simulink model "Controller"  (R2015b)
settings: Solver=FixedStepAuto  StartTime=0.0  StopTime=inf  FixedStep=0.1  RelTol=1e-3
InitFcn:
  | robotics.ros.createSimulinkBus(gcs);
model workspace (MAT data in the model file):
  SL_ROS_VariableLengthArrays_MaxSizes : struct (value not decoded)
undefined symbols (not defined in the file or in its folder): DiscIntNeverNeededParam
libraries: robotlib x66, simulink x7, dspsrcs4 x6
(part 2 of 2)

== system Controller/toPWM/Enable thrusters  ==
  Get Parameter : robotlib/Get Parameter  SourceLibraryInfo=This block requires Robotics System Toolbox  ParameterSource=Specify your own  ParameterName=/matlab_controller/enable_thruster1  ParameterType=boolean  ParameterInitialValue=1  SampleTime=-1  ShowErrorCodeOutput=off  ModelName=Controller_without_ref  BlockId=ParamGet_Controller_without_ref_858
  Get Parameter1 : robotlib/Get Parameter  SourceLibraryInfo=This block requires Robotics System Toolbox  ParameterSource=Specify your own  ParameterName=/matlab_controller/enable_thruster2  ParameterType=boolean  ParameterInitialValue=1  SampleTime=-1  ShowErrorCodeOutput=off  ModelName=Controller_without_ref  BlockId=ParamGet_Controller_without_ref_861
  Get Parameter2 : robotlib/Get Parameter  SourceLibraryInfo=This block requires Robotics System Toolbox  ParameterSource=Specify your own  ParameterName=/matlab_controller/enable_thruster3  ParameterType=boolean  ParameterInitialValue=1  SampleTime=-1  ShowErrorCodeOutput=off  ModelName=Controller_without_ref  BlockId=ParamGet_Controller_without_ref_862
  Get Parameter3 : robotlib/Get Parameter  SourceLibraryInfo=This block requires Robotics System Toolbox  ParameterSource=Specify your own  ParameterName=/matlab_controller/enable_thruster4  ParameterType=boolean  ParameterInitialValue=1  SampleTime=-1  ShowErrorCodeOutput=off  ModelName=Controller_without_ref  BlockId=ParamGet_Controller_without_ref_863
  Get Parameter4 : robotlib/Get Parameter  SourceLibraryInfo=This block requires Robotics System Toolbox  ParameterSource=Specify your own  ParameterName=/matlab_controller/enable_thruster5  ParameterType=boolean  ParameterInitialValue=1  SampleTime=-1  ShowErrorCodeOutput=off  ModelName=Controller_without_ref  BlockId=ParamGet_Controller_without_ref_864
  Get Parameter5 : robotlib/Get Parameter  SourceLibraryInfo=This block requires Robotics System Toolbox  ParameterSource=Specify your own  ParameterName=/matlab_controller/enable_thruster6  ParameterType=boolean  ParameterInitialValue=1  SampleTime=-1  ShowErrorCodeOutput=off  ModelName=Controller_without_ref  BlockId=ParamGet_Controller_without_ref_865
  Mux : Mux  Inputs=6
  enable_thrusters : Outport
  wires:
  Get Parameter/1 -> Mux/1
  Get Parameter1/1 -> Mux/2
  Get Parameter2/1 -> Mux/3
  Get Parameter3/1 -> Mux/4
  Get Parameter4/1 -> Mux/5
  Get Parameter5/1 -> Mux/6
  Mux/1 -> enable_thrusters/1

== system Controller/decController/angular_vel x/Retrive PID-Parameters ==
  D_angular_vel_x : robotlib/Get Parameter  SourceLibraryInfo=This block requires Robotics System Toolbox  ParameterSource=Select from ROS network  ParameterName=/matlab_controller/D_angular_vel_x  ParameterType=double  ParameterInitialValue=0  SampleTime=-1  ShowErrorCodeOutput=off  ModelName=Controller_without_ref  BlockId=ParamGet_Controller_without_ref_505
  I_angular_vel_x : robotlib/Get Parameter  SourceLibraryInfo=This block requires Robotics System Toolbox  ParameterSource=Select from ROS network  ParameterName=/matlab_controller/I_angular_vel_x  ParameterType=double  ParameterInitialValue=0  SampleTime=-1  ShowErrorCodeOutput=off  ModelName=Controller_without_ref  BlockId=ParamGet_Controller_without_ref_506
  "N_angular_vel_x " : robotlib/Get Parameter  SourceLibraryInfo=This block requires Robotics System Toolbox  ParameterSource=Specify your own  ParameterName=/matlab_controller/N_angular_vel_x  ParameterType=double  ParameterInitialValue=0  SampleTime=-1  ShowErrorCodeOutput=off  ModelName=Controller_without_ref  BlockId=ParamGet_Controller_without_ref_507
  P_angular_vel_x : robotlib/Get Parameter  SourceLibraryInfo=This block requires Robotics System Toolbox  ParameterSource=Select from ROS network  ParameterName=/matlab_controller/P_angular_vel_x  ParameterType=double  ParameterInitialValue=0  SampleTime=-1  ShowErrorCodeOutput=off  ModelName=Controller_without_ref  BlockId=ParamGet_Controller_without_ref_508
  P : Outport
  I : Outport  Port=2
  D : Outport  Port=3
  N : Outport  Port=4
  wires:
  "N_angular_vel_x "/1 -> N/1
  D_angular_vel_x/1 -> D/1
  I_angular_vel_x/1 -> I/1
  P_angular_vel_x/1 -> P/1

== system Controller/decController/angular_vel y/Retrive PID-Parameters ==
  D_angular_vel_y : robotlib/Get Parameter  SourceLibraryInfo=This block requires Robotics System Toolbox  ParameterSource=Specify your own  ParameterName=/matlab_controller/D_angular_vel_y  ParameterType=double  ParameterInitialValue=0  SampleTime=-1  ShowErrorCodeOutput=off  ModelName=Controller_without_ref  BlockId=ParamGet_Controller_without_ref_519
  I_angular_vel_y : robotlib/Get Parameter  SourceLibraryInfo=This block requires Robotics System Toolbox  ParameterSource=Specify your own  ParameterName=/matlab_controller/I_angular_vel_y  ParameterType=double  ParameterInitialValue=0  SampleTime=-1  ShowErrorCodeOutput=off  ModelName=Controller_without_ref  BlockId=ParamGet_Controller_without_ref_520
  "N_angular_vel_y " : robotlib/Get Parameter  SourceLibraryInfo=This block requires Robotics System Toolbox  ParameterSource=Specify your own  ParameterName=/matlab_controller/N_angular_vel_y  ParameterType=double  ParameterInitialValue=0  SampleTime=-1  ShowErrorCodeOutput=off  ModelName=Controller_without_ref  BlockId=ParamGet_Controller_without_ref_521
  P_angular_vel_y : robotlib/Get Parameter  SourceLibraryInfo=This block requires Robotics System Toolbox  ParameterSource=Specify your own  ParameterName=/matlab_controller/P_angular_vel_y  ParameterType=double  ParameterInitialValue=0  SampleTime=-1  ShowErrorCodeOutput=off  ModelName=Controller_without_ref  BlockId=ParamGet_Controller_without_ref_522
  P : Outport
  I : Outport  Port=2
  D : Outport  Port=3
  N : Outport  Port=4
  wires:
  "N_angular_vel_y "/1 -> N/1
  D_angular_vel_y/1 -> D/1
  I_angular_vel_y/1 -> I/1
  P_angular_vel_y/1 -> P/1

== system Controller/decController/angular_vel z/Retrive PID-Parameters ==
  D_angular_vel_z : robotlib/Get Parameter  SourceLibraryInfo=This block requires Robotics System Toolbox  ParameterSource=Specify your own  ParameterName=/matlab_controller/D_angular_vel_z  ParameterType=double  ParameterInitialValue=0  SampleTime=-1  ShowErrorCodeOutput=off  ModelName=Controller_without_ref  BlockId=ParamGet_Controller_without_ref_533
  I_angular_vel_z : robotlib/Get Parameter  SourceLibraryInfo=This block requires Robotics System Toolbox  ParameterSource=Specify your own  ParameterName=/matlab_controller/I_angular_vel_z  ParameterType=double  ParameterInitialValue=0  SampleTime=-1  ShowErrorCodeOutput=off  ModelName=Controller_without_ref  BlockId=ParamGet_Controller_without_ref_534
  "N_angular_vel_z " : robotlib/Get Parameter  SourceLibraryInfo=This block requires Robotics System Toolbox  ParameterSource=Specify your own  ParameterName=/matlab_controller/N_angular_vel_z  ParameterType=double  ParameterInitialValue=0  SampleTime=-1  ShowErrorCodeOutput=off  ModelName=Controller_without_ref  BlockId=ParamGet_Controller_without_ref_535
  P_angular_vel_z : robotlib/Get Parameter  SourceLibraryInfo=This block requires Robotics System Toolbox  ParameterSource=Specify your own  ParameterName=/matlab_controller/P_angular_vel_z  ParameterType=double  ParameterInitialValue=0  SampleTime=-1  ShowErrorCodeOutput=off  ModelName=Controller_without_ref  BlockId=ParamGet_Controller_without_ref_536
  P : Outport
  I : Outport  Port=2
  D : Outport  Port=3
  N : Outport  Port=4
  wires:
  "N_angular_vel_z "/1 -> N/1
  D_angular_vel_z/1 -> D/1
  I_angular_vel_z/1 -> I/1
  P_angular_vel_z/1 -> P/1

== system Controller/decController/vel x/Retrive PID-Parameters ==
  D_vel_x : robotlib/Get Parameter  SourceLibraryInfo=This block requires Robotics System Toolbox  ParameterSource=Specify your own  ParameterName=/matlab_controller/D_vel_x  ParameterType=double  ParameterInitialValue=0  SampleTime=-1  ShowErrorCodeOutput=off  ModelName=Controller_without_ref  BlockId=ParamGet_Controller_without_ref_547
  I_vel_x : robotlib/Get Parameter  SourceLibraryInfo=This block requires Robotics System Toolbox  ParameterSource=Specify your own  ParameterName=/matlab_controller/I_vel_x  ParameterType=double  ParameterInitialValue=0  SampleTime=-1  ShowErrorCodeOutput=off  ModelName=Controller_without_ref  BlockId=ParamGet_Controller_without_ref_548
  "N_vel_x " : robotlib/Get Parameter  SourceLibraryInfo=This block requires Robotics System Toolbox  ParameterSource=Specify your own  ParameterName=/matlab_controller/N_vel_x  ParameterType=double  ParameterInitialValue=0  SampleTime=-1  ShowErrorCodeOutput=off  ModelName=Controller_without_ref  BlockId=ParamGet_Controller_without_ref_549
  P_vel_x : robotlib/Get Parameter  SourceLibraryInfo=This block requires Robotics System Toolbox  ParameterSource=Specify your own  ParameterName=/matlab_controller/P_vel_x  ParameterType=double  ParameterInitialValue=0  SampleTime=-1  ShowErrorCodeOutput=off  ModelName=Controller_without_ref  BlockId=ParamGet_Controller_without_ref_550
  P : Outport
  I : Outport  Port=2
  D : Outport  Port=3
  N : Outport  Port=4
  wires:
  "N_vel_x "/1 -> N/1
  D_vel_x/1 -> D/1
  I_vel_x/1 -> I/1
  P_vel_x/1 -> P/1

== system Controller/decController/vel y/Retrive PID-Parameters ==
  D_vel_y : robotlib/Get Parameter  SourceLibraryInfo=This block requires Robotics System Toolbox  ParameterSource=Specify your own  ParameterName=/matlab_controller/D_vel_y  ParameterType=double  ParameterInitialValue=0  SampleTime=-1  ShowErrorCodeOutput=off  ModelName=Controller_without_ref  BlockId=ParamGet_Controller_without_ref_561
  I_vel_y : robotlib/Get Parameter  SourceLibraryInfo=This block requires Robotics System Toolbox  ParameterSource=Specify your own  ParameterName=/matlab_controller/I_vel_y  ParameterType=double  ParameterInitialValue=0  SampleTime=-1  ShowErrorCodeOutput=off  ModelName=Controller_without_ref  BlockId=ParamGet_Controller_without_ref_562
  "N_vel_y " : robotlib/Get Parameter  SourceLibraryInfo=This block requires Robotics System Toolbox  ParameterSource=Specify your own  ParameterName=/matlab_controller/N_vel_y  ParameterType=double  ParameterInitialValue=0  SampleTime=-1  ShowErrorCodeOutput=off  ModelName=Controller_without_ref  BlockId=ParamGet_Controller_without_ref_563
  P_vel_y : robotlib/Get Parameter  SourceLibraryInfo=This block requires Robotics System Toolbox  ParameterSource=Specify your own  ParameterName=/matlab_controller/P_vel_y  ParameterType=double  ParameterInitialValue=0  SampleTime=-1  ShowErrorCodeOutput=off  ModelName=Controller_without_ref  BlockId=ParamGet_Controller_without_ref_564
  P : Outport
  I : Outport  Port=2
  D : Outport  Port=3
  N : Outport  Port=4
  wires:
  "N_vel_y "/1 -> N/1
  D_vel_y/1 -> D/1
  I_vel_y/1 -> I/1
  P_vel_y/1 -> P/1

== system Controller/decController/vel z/Retrive PID-Parameters ==
  D_vel_z : robotlib/Get Parameter  SourceLibraryInfo=This block requires Robotics System Toolbox  ParameterSource=Specify your own  ParameterName=/matlab_controller/D_vel_z  ParameterType=double  ParameterInitialValue=0  SampleTime=-1  ShowErrorCodeOutput=off  ModelName=Controller_without_ref  BlockId=ParamGet_Controller_without_ref_575
  I_vel_z : robotlib/Get Parameter  SourceLibraryInfo=This block requires Robotics System Toolbox  ParameterSource=Specify your own  ParameterName=/matlab_controller/I_vel_z  ParameterType=double  ParameterInitialValue=0  SampleTime=-1  ShowErrorCodeOutput=off  ModelName=Controller_without_ref  BlockId=ParamGet_Controller_without_ref_576
  "N_vel_z " : robotlib/Get Parameter  SourceLibraryInfo=This block requires Robotics System Toolbox  ParameterSource=Specify your own  ParameterName=/matlab_controller/N_vel_z  ParameterType=double  ParameterInitialValue=0  SampleTime=-1  ShowErrorCodeOutput=off  ModelName=Controller_without_ref  BlockId=ParamGet_Controller_without_ref_577
  P_vel_z : robotlib/Get Parameter  SourceLibraryInfo=This block requires Robotics System Toolbox  ParameterSource=Specify your own  ParameterName=/matlab_controller/P_vel_z  ParameterType=double  ParameterInitialValue=0  SampleTime=-1  ShowErrorCodeOutput=off  ModelName=Controller_without_ref  BlockId=ParamGet_Controller_without_ref_578
  P : Outport
  I : Outport  Port=2
  D : Outport  Port=3
  N : Outport  Port=4
  wires:
  "N_vel_z "/1 -> N/1
  D_vel_z/1 -> D/1
  I_vel_z/1 -> I/1
  P_vel_z/1 -> P/1

== matlab function Controller/Telegraph/Thruster1 block/MATLAB Function ==
  data: u input; y output; min_scale input; max_scale input
function y = fcn(u,min_scale,max_scale)
%#codegen
    
    if (u < 0)
        y = min_scale*u;
    else
        y = max_scale*u;
    end
end

== matlab function Controller/Decouple2/MATLAB Function ==
  data: angular_x input; thruster1 output; angular_y input; angular_z input; vel_x input; vel_y input; vel_z input; front_strafe_decouple input; front_forward_decouple input; front_pitch_bias input; front_vertical_bias input; buoyancy_control input; thruster2 output; thruster3 output; thruster4 output; thruster5 output; thruster6 output
function [thruster1,thruster2,thruster3,thruster4,thruster5,thruster6] =...
    basicdecouple(angular_x,angular_y,angular_z,vel_x,vel_y,vel_z,...
    front_strafe_decouple,front_forward_decouple,front_pitch_bias,...
    front_vertical_bias,buoyancy_control)

% Vertical Left thruster (VL)
thruster1 =...
    angular_x...
    -front_forward_decouple*vel_x...
    -front_strafe_decouple*vel_y...
    -front_pitch_bias*angular_y...
    +front_vertical_bias*vel_z...
    +buoyancy_control; 


% Vertical Back thruster (VB)
thruster2 =...
    front_forward_decouple * vel_x...
    +angular_y...
    +vel_z...
    +buoyancy_control; 


thruster3 =...
    -angular_x...
    -front_forward_decouple * vel_x+...
    front_strafe_decouple*vel_y...
    -front_pitch_bias*angular_y...
    +front_vertical_bias * vel_z...
    +buoyancy_control;

 %Forward Left (FL)
thruster4 =...
    -angular_z...
    + vel_x;
thruster5 = vel_y; % LATeral (LAT)

% Forward Right (FR)
thruster6 =...
    angular_z...
    + vel_x;

end

== matlab function Controller/states/removeGravity ==
  data: yaw input; pitch input; roll input; x_acc input; y_acc input; z_acc input; x_accnew output; y_accnew output; z_accnew output
function [x_accnew,y_accnew,z_accnew]  = removeGravity(yaw,pitch,roll,x_acc,y_acc,z_acc)
%#codegen

% rotmatrix = [2*w^2+2*x^2-1, 2*x*y-2*w*z, 2*x*z+2*w*y; 
%     2*x*y+2*w*z, 2*w^2+2*y^2-1, 2*x*z-2*w*x;
%     2*x*z-2*w*y, 2*y*z+2*w*x, 2*w^2+2*z^2-1];

sfi = sind(roll);
cfi = cosd(roll);
spsi = sind(yaw);
cpsi = cosd(yaw);
stheta = sind(pitch);
ctheta = cosd(pitch);


rotmatrix = ([...
    cpsi(i)*ctheta(i), -spsi(i)*cfi(i)+cpsi(i)*stheta(i)*sfi(i), spsi(i)*sfi(i)+cpsi(i)*cfi(i)*stheta(i);
    spsi(i)*ctheta(i), cpsi(i)*cfi(i)+sfi(i)*stheta(i)*spsi(i), -cpsi(i)*sfi(i)+stheta(i)*spsi(i)*cfi(i);
    -stheta(i), ctheta(i)*sfi(i), ctheta(i)*cfi(i)].');

g = [0;0;9.80];
% Gravity projected in the body fixed frame
acc = rotmatrix*g;

% Removed gravity from the acceleration
x_accnew = x_acc+acc(1);
y_accnew = y_acc+acc(2);
z_accnew = z_acc+acc(3);
end

== matlab function Controller/toPWM/Calc pwm signal ==
  data: controlsignal input; pwm output
function pwm = calcPWM(controlsignal)
 % thruster values should be between 1100 and 1900 microseconds (us)
 % values less than 1500 us are backwards; values more than are forwards

pwm=(controlsignal + 1) * 400 + 1100;

end

== matlab function Controller/toPWM/PWM assign ==
  data: blankMessage input Bus: SL_Bus_Controller_without_ref_std_msgs_UInt16MultiArray; data input size=6; msg output Bus: SL_Bus_Controller_without_ref_std_msgs_UInt16MultiArray
function msg = assignArray(blankMessage,data)
%#codegen

blankMessage.Data = data;
blankMessage.Layout.DataOffset = uint32(0);
blankMessage.Layout.Dim(1).Stride = uint32(1);
blankMessage.Layout.Dim(1).Size = uint32(6);
blankMessage.Data_SL_Info.CurrentLength = uint32(6);
msg = blankMessage;

end

== stateflow chart Controller/Telegraph/Thruster1 block/State Transition Table ==
  state state1
  state state2
  (default) -> state1
  state1 -> (junction 20) [order 2]
  (junction 20) -> state1
  state1 -> state2 [order 1] : [x > 0]
      | {u = 1}
  state2 -> state1 [order 1] : [x> 0]
      | {u= -1}
  state2 -> (junction 24) [order 2]
  (junction 24) -> state2
  data: x input; u output

== matlab function Controller/Telegraph/Thruster2 block/MATLAB Function ==
  data: u input; y output; min_scale input; max_scale input
function y = fcn(u,min_scale,max_scale)
%#codegen
    
    if (u < 0)
        y = min_scale*u;
    else
        y = max_scale*u;
    end
end

== stateflow chart Controller/Telegraph/Thruster2 block/State Transition Table ==
  state state1
  state state2
  (default) -> state1
  state1 -> (junction 20) [order 2]
  (junction 20) -> state1
  state1 -> state2 [order 1] : [x > 0]
      | {u = 1}
  state2 -> state1 [order 1] : [x> 0]
      | {u= -1}
  state2 -> (junction 24) [order 2]
  (junction 24) -> state2
  data: x input; u output

== matlab function Controller/Telegraph/Thruster3 block/MATLAB Function ==
  data: u input; y output; min_scale input; max_scale input
function y = fcn(u,min_scale,max_scale)
%#codegen
    
    if (u < 0)
        y = min_scale*u;
    else
        y = max_scale*u;
    end
end

== stateflow chart Controller/Telegraph/Thruster3 block/State Transition Table ==
  state state1
  state state2
  (default) -> state1
  state1 -> (junction 20) [order 2]
  (junction 20) -> state1
  state1 -> state2 [order 1] : [x > 0]
      | {u = 1}
  state2 -> state1 [order 1] : [x> 0]
      | {u= -1}
  state2 -> (junction 24) [order 2]
  (junction 24) -> state2
  data: x input; u output

== matlab function Controller/Telegraph/Thruster4 block/MATLAB Function ==
  data: u input; y output; min_scale input; max_scale input
function y = fcn(u,min_scale,max_scale)
%#codegen
    
    if (u < 0)
        y = min_scale*u;
    else
        y = max_scale*u;
    end
end

== stateflow chart Controller/Telegraph/Thruster4 block/State Transition Table ==
  state state1
  state state2
  (default) -> state1
  state1 -> (junction 20) [order 2]
  (junction 20) -> state1
  state1 -> state2 [order 1] : [x > 0]
      | {u = 1}
  state2 -> state1 [order 1] : [x> 0]
      | {u= -1}
  state2 -> (junction 24) [order 2]
  (junction 24) -> state2
  data: x input; u output

== matlab function Controller/Telegraph/Thruster5 block /MATLAB Function ==
  data: u input; y output; min_scale input; max_scale input
function y = fcn(u,min_scale,max_scale)
%#codegen
    
    if (u < 0)
        y = min_scale*u;
    else
        y = max_scale*u;
    end
end

== stateflow chart Controller/Telegraph/Thruster5 block /State Transition Table ==
  state state1
  state state2
  (default) -> state1
  state1 -> (junction 20) [order 2]
  (junction 20) -> state1
  state1 -> state2 [order 1] : [x > 0]
      | {u = 1}
  state2 -> state1 [order 1] : [x> 0]
      | {u= -1}
  state2 -> (junction 24) [order 2]
  (junction 24) -> state2
  data: x input; u output

== matlab function Controller/Telegraph/Thruster6 block/MATLAB Function ==
  data: u input; y output; min_scale input; max_scale input
function y = fcn(u,min_scale,max_scale)
%#codegen
    
    if (u < 0)
        y = min_scale*u;
    else
        y = max_scale*u;
    end
end

== stateflow chart Controller/Telegraph/Thruster6 block/State Transition Table ==
  state state1
  state state2
  (default) -> state1
  state1 -> (junction 20) [order 2]
  (junction 20) -> state1
  state1 -> state2 [order 1] : [x > 0]
      | {u = 1}
  state2 -> state1 [order 1] : [x> 0]
      | {u= -1}
  state2 -> (junction 24) [order 2]
  (junction 24) -> state2
  data: x input; u output

== matlab function Controller/Decouple1/MATLAB Function ==
  data: angular_x input; thruster1 output; angular_y input; angular_z input; vel_x input; vel_y input; vel_z input; front_strafe_decouple input; front_forward_decouple input; front_pitch_bias input; front_vertical_bias input; buoyancy_control input; thruster2 output; thruster3 output; thruster4 output; thruster5 output; thruster6 output
function [thruster1,thruster2,thruster3,thruster4,thruster5,thruster6] =...
    basicdecouple(angular_x,angular_y,angular_z,vel_x,vel_y,vel_z,...
    front_strafe_decouple,front_forward_decouple,front_pitch_bias,...
    front_vertical_bias,buoyancy_control)

% Vertical Left thruster (VL)
thruster1 =...
    angular_x...
    -front_forward_decouple*vel_x...
    -front_strafe_decouple*vel_y...
    -front_pitch_bias*angular_y...
    +front_vertical_bias*vel_z...
    +buoyancy_control; 


% Vertical Back thruster (VB)
thruster2 =...
    front_forward_decouple * vel_x...
    +angular_y...
    +vel_z...
    +buoyancy_control; 


thruster3 =...
    -angular_x...
    -front_forward_decouple * vel_x+...
    front_strafe_decouple*vel_y...
    -front_pitch_bias*angular_y...
    +front_vertical_bias * vel_z...
    +buoyancy_control;

 %Forward Left (FL)
thruster4 =...
    -angular_z...
    + vel_x;
thruster5 = vel_y; % LATeral (LAT)

% Forward Right (FR)
thruster6 =...
    angular_z...
    + vel_x;

end
